simulink model "real_time_2_4"  (R2022b)
settings: Solver=FixedStepAuto  StartTime=0.0  StopTime=inf  RelTol=1e-3
undefined symbols (not defined in the file or in its folder): Serial_Port, Standard_Devices
libraries: sldrtlib x2
settings Model: SimulationMode=external  Creator=bdjdkn  LastModifiedBy=bdjdkn
settings SolverCC: AlgebraicLoopSolver=TrustRegion  AutoInsertRateTranBlk=on  DecoupledContinuousIntegration=on  MinimalZcImpactIntegration=on
settings DataIOCC: ReturnWorkspaceOutputs=off
settings DebuggingCC: UnconnectedInputMsg=warning  UnconnectedOutputMsg=warning  UnconnectedLineMsg=warning  SFMachineParentedDataDiag=warning  ArithmeticOperatorsInVariantConditions=warning
settings HardwareCC: ProdBitPerLong=64  ProdHWDeviceType=Intel->x86-64 (Linux 64)
settings ModelReferenceCC: EnableRefExpFcnMdlSchedulingChecks=on
settings SFSimCC: SimUseLocalCustomCode=off  CustomCodeUndefinedFunction=UseInterfaceOnly
settings RTWCC: Description=Simulink Desktop Real-Time  SystemTargetFile=sldrt.tlc  TemplateMakefile=sldrt.tmf  RTWUseLocalCustomCode=off  RTWCompilerOptimization=on  DLArmComputeVersion=19.05
settings CodeAppCC: MaxIdLength=95
settings SimulinkDesktopRealTimeCC: TargetLibSuffix=_sldrt.a  TargetPreCompLibLocation=C:\Program Files\MATLAB\R2022b\toolbox\sldrt\lib\win64

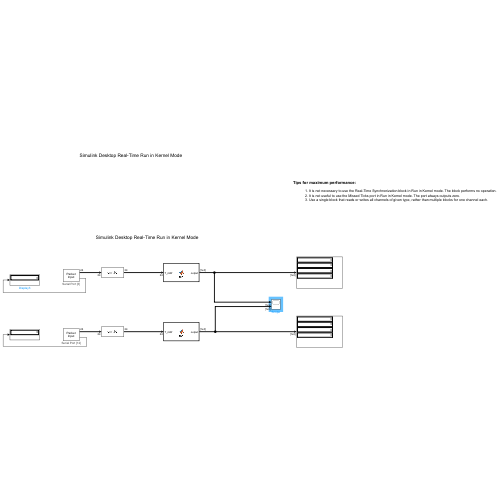
[thumbnail: Simulink's stored preview of the top-level diagram]
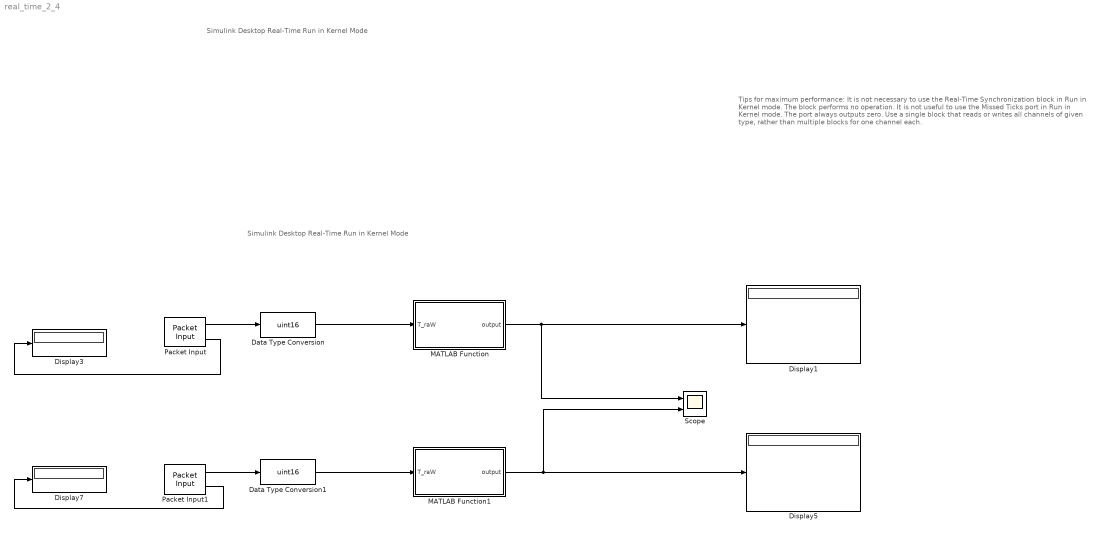
== system real_time_2_4 ==
  note: Tips for maximum performance:
      |
      | It is not necessary to use the Real-Time Synchronization block in Run in Kernel mode. The block performs no operation.
      | It is not useful to use the Missed Ticks port in Run in Kernel mode. The port always outputs zero.
      | Use a single block that reads or writes all channels of given type, rather than multiple blocks for one channel each.
  note: Simulink Desktop Real-Time Run in Kernel Mode
  note: Simulink Desktop Real-Time Run in Kernel Mode
  Data Type Conversion : DataTypeConversion  OutDataTypeStr=uint16  SaturateOnIntegerOverflow=off  RndMeth=Floor
  Data Type Conversion1 : DataTypeConversion  OutDataTypeStr=uint16  SaturateOnIntegerOverflow=off  RndMeth=Floor
  Display{1,3,5,7} (4 alike) : Display
      Display3 settings: Format=decimal (Stored Integer)
      Display7 settings: Format=decimal (Stored Integer)
  MATLAB Function : MATLAB Function  TreatAsAtomicUnit=on
  MATLAB Function1 : MATLAB Function  TreatAsAtomicUnit=on
  Packet Input : sldrtlib/Packet Input  SampleTime=0.002  MaxMissedTicks=100000000  ShowMissedTicks=on  YieldWhenWaiting=off  DrvName=Standard_Devices/Serial_Port  DrvAddress=3  DrvOptions=[115200 8 0 0 0 0 0 1]  PacketSize=24  DataTypes='24*uint8'  ShowReady=off  ShowError=off  PacketID=1  ByteOrder=1  ShowTimestamp=off
      settings: AttributesFormatString=Serial Port [3]
  Packet Input1 : sldrtlib/Packet Input  SampleTime=0.002  MaxMissedTicks=100000000  ShowMissedTicks=on  YieldWhenWaiting=off  DrvName=Standard_Devices/Serial_Port  DrvAddress=12  DrvOptions=[115200 8 0 0 0 0 0 0]  PacketSize=24  DataTypes='24*uint8'  ShowReady=off  ShowError=off  PacketID=1  ByteOrder=1  ShowTimestamp=off
      settings: AttributesFormatString=Serial Port [12]
  Scope : Scope  NumInputPorts=2
  wires:
  MATLAB Function/1(output) -> Display1/1, Scope/1
  Packet Input/2 -> Display3/1
  Packet Input/1 -> Data Type Conversion/1
  Data Type Conversion/1 -> MATLAB Function/1(T_raW)
  Packet Input1/1 -> Data Type Conversion1/1
  Packet Input1/2 -> Display7/1
  MATLAB Function1/1(output) -> Scope/2, Display5/1
  Data Type Conversion1/1 -> MATLAB Function1/1(T_raW)

== matlab function real_time_2_4/MATLAB Function1 ==
  data: T_raW input; output output int64
function output= fcn(T_raW)
%%%%%%%%%%%%%%%%%%%%%%%%%
%数据初始化
t_uint32=uint32([0,0,0,0]);%uint32型原始数据，无正负
t_int32=int64([0,0,0,0]);%加了负号后的真正数据
y=[T_raW ,T_raW];%由于MATLAB不支持指针进行首尾相连，所以两个数据和一块类似首尾相连，应对帧头不在第一位的问题
flag_star=-1;%帧头的标志
channel=4;%通道数
%%%%%%%%%%%%%%%%%%%%%%%%%
%判断帧头的位置
for i=1:8+channel*4
    
    if y(i)==254
        flag_star=i;
    end
end
%%%%%%%%%%%%%%%%%%%%%%%%%
%判断帧尾的位置
if flag_star~=-1&&y(flag_star+channel*4+4)==207&&y(flag_star+channel*4+5)==252&&y(flag_star+channel*4+6)==204&&y(flag_star+channel*4+7)==255
    for i=1:channel
        %循环读取数据
        data=[0,0,0,0];
        data(1)=y(flag_star+i*4);
        data(2)=y(flag_star+i*4+1);
        data(3)=y(flag_star+i*4+2);
        data(4)=y(flag_star+i*4+3);
        %进制转换   依次为16^0,16^2,16^4,16^6
        t_uint32(i)=uint32( data(1)*16777216+data(2)*65536+data(3)*256+data(4));
        %转换为int32类型，判断正负
        if t_uint32(i)>4000000000
            t_int32(i)=int64(t_uint32(i))-4294967295;
        else
            t_int32(i)=int64(t_uint32(i));
        end
    end
end
%最终输出
output=t_int32;
end

== matlab function real_time_2_4/MATLAB Function ==
  data: T_raW input; output output int64
function output= fcn(T_raW)
%%%%%%%%%%%%%%%%%%%%%%%%%
%数据初始化
t_uint32=uint32([0,0,0,0]);%uint32型原始数据，无正负
t_int32=int64([0,0,0,0]);%加了负号后的真正数据
y=[T_raW ,T_raW];%由于MATLAB不支持指针进行首尾相连，所以两个数据和一块类似首尾相连，应对帧头不在第一位的问题
flag_star=-1;%帧头的标志
channel=4;%通道数
%%%%%%%%%%%%%%%%%%%%%%%%%
%判断帧头的位置
for i=1:8+channel*4
    
    if y(i)==254
        flag_star=i;
    end
end
%%%%%%%%%%%%%%%%%%%%%%%%%
%判断帧尾的位置
if flag_star~=-1&&y(flag_star+channel*4+4)==207&&y(flag_star+channel*4+5)==252&&y(flag_star+channel*4+6)==204&&y(flag_star+channel*4+7)==255
    for i=1:channel
        %循环读取数据
        data=[0,0,0,0];
        data(1)=y(flag_star+i*4);
        data(2)=y(flag_star+i*4+1);
        data(3)=y(flag_star+i*4+2);
        data(4)=y(flag_star+i*4+3);
        %进制转换   依次为16^0,16^2,16^4,16^6
        t_uint32(i)=uint32( data(1)*16777216+data(2)*65536+data(3)*256+data(4));
        %转换为int32类型，判断正负
        if t_uint32(i)>4000000000
            t_int32(i)=int64(t_uint32(i))-4294967295;
        else
            t_int32(i)=int64(t_uint32(i));
        end
    end
end
%最终输出
output=t_int32;
end
